simulink model "ImpactVelocityFunction"  (R2019a)
settings: Solver=FixedStepAuto  StartTime=0.0  StopTime=20  FixedStep=0.00001  RelTol=1e-5  AbsTol=1e-8
PostLoadFcn:
  | ThrustTable = xlsread('F15_Thrust','Sheet1');
settings Model: SimulationMode=accelerator  Creator=rag  LastModifiedBy=rag

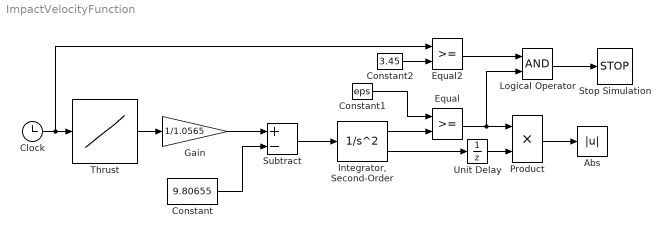
== system ImpactVelocityFunction ==
  Abs : Abs
  Clock : Clock
  Constant : Constant  Value=9.80655
  Constant1 : Constant  Value=eps
  Constant2 : Constant  Value=3.45
  Equal : RelationalOperator  OutDataTypeStr=boolean  RndMeth=Simplest
  Equal2 : RelationalOperator  OutDataTypeStr=boolean  RndMeth=Simplest
  Gain : Gain  Gain=1/1.0565
  "Integrator, Second-Order" : SecondOrderIntegrator  ICX=s0  LimitX=on  LowerLimitX=0  ICDXDT=v0
  Logical Operator : Logic  AllPortsSameDT=off  OutDataTypeStr=boolean
  Product : Product
  Stop Simulation : Stop
  Subtract : Sum  Inputs=+-
  Thrust : Lookup_n-D  NumberOfTableDimensions=1  BreakpointsForDimension1=ThrustTable(:,1)  BreakpointsForDimension1FirstPoint=0  BreakpointsForDimension1Spacing=1.5e-5  Table=ThrustTable(:,2)  ExtrapMethod=Clip  InternalRulePriority=Speed  RndMeth=Simplest  InputSameDT=on
  Unit Delay : UnitDelay  SampleTime=-1  HasFrameUpgradeWarning=on
  wires:
  Thrust/1 -> Gain/1
  Gain/1 -> Subtract/1
  Constant/1 -> Subtract/2
  Clock/1 -> Equal2/1, Thrust/1
  Subtract/1 -> "Integrator, Second-Order"/1
  "Integrator, Second-Order"/1 -> Equal/2
  "Integrator, Second-Order"/2 -> Unit Delay/1
  Constant1/1 -> Equal/1
  Product/1 -> Abs/1
  Equal/1 -> Logical Operator/2, Product/1
  Unit Delay/1 -> Product/2
  Equal2/1 -> Logical Operator/1
  Logical Operator/1 -> Stop Simulation/1
  Constant2/1 -> Equal2/2
